simulink model "MappedCornerStiffness"  (R2021a)
settings: Solver=VariableStepAuto  StartTime=0.0  StopTime=15  RelTol=1e-3
values from neighbouring files (symbols this model uses):
  Ts = 0.05    [controller_setup.m]    (also in test.m = 0.1)
libraries: autolibshared x4
settings Model: Creator=chnwa  LastModifiedBy=chnwa

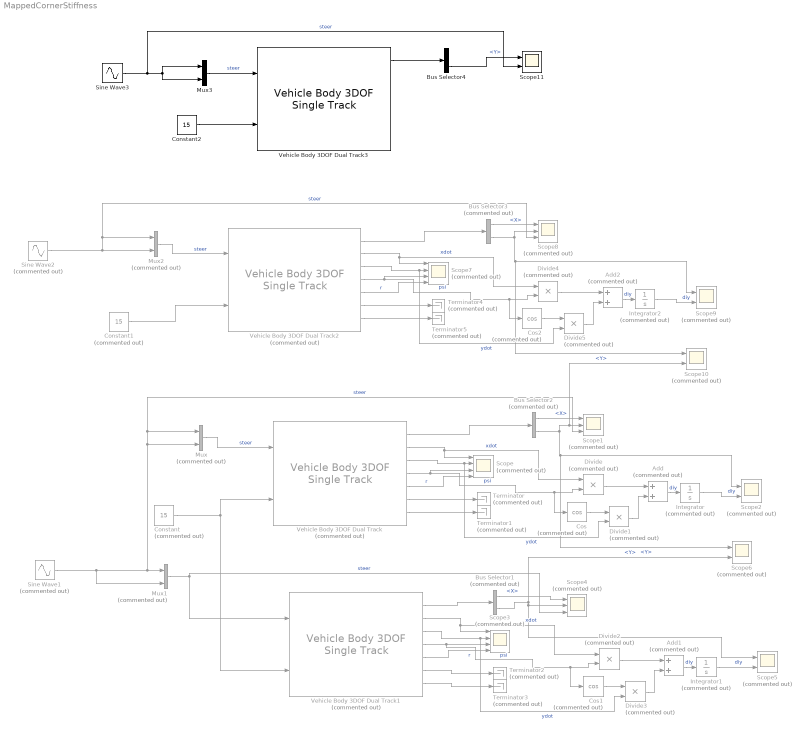
== system MappedCornerStiffness ==
  Add : Sum  Commented=on
  Add1 : Sum  Commented=on
  Add2 : Sum  Commented=on
  Bus Selector1 : BusSelector  Commented=on  OutputSignals=InertFrm.Cg.Disp.X,InertFrm.Cg.Disp.Y
  Bus Selector2 : BusSelector  Commented=on  OutputSignals=InertFrm.Cg.Disp.X,InertFrm.Cg.Disp.Y
  Bus Selector3 : BusSelector  Commented=on  OutputSignals=InertFrm.Cg.Disp.X,InertFrm.Cg.Disp.Y
  Bus Selector4 : BusSelector  OutputSignals=InertFrm.Cg.Disp.X,InertFrm.Cg.Disp.Y
  Constant : Constant  Commented=on  Value=15
  Constant1 : Constant  Commented=on  Value=15
  Constant2 : Constant  Value=15
  Cos : Trigonometry  Commented=on  Operator=cos
  Cos1 : Trigonometry  Commented=on  Operator=cos
  Cos2 : Trigonometry  Commented=on  Operator=cos
  Divide{,1..5} (6 alike) : Product  Commented=on  Inputs=**
  Integrator : Integrator  Commented=on
  Integrator1 : Integrator  Commented=on
  Integrator2 : Integrator  Commented=on
  Mux : Mux  Commented=on  Inputs=2
  Mux1 : Mux  Commented=on  Inputs=2
  Mux2 : Mux  Commented=on  Inputs=2
  Mux3 : Mux  Inputs=2
  Scope : Scope  Commented=on  NumInputPorts=4
  Scope1 : Scope  Commented=on  NumInputPorts=3
  Scope{2,5..6,9..10} (5 alike) : Scope  Commented=on  NumInputPorts=2
  Scope11 : Scope  NumInputPorts=2
  Scope3 : Scope  Commented=on  NumInputPorts=4
  Scope4 : Scope  Commented=on  NumInputPorts=3
  Scope7 : Scope  Commented=on  NumInputPorts=4
  Scope8 : Scope  Commented=on  NumInputPorts=3
  Sine Wave1 : Sin  Commented=on  Amplitude=0.01  Frequency=pi/5  SampleTime=Ts
  Sine Wave2 : Sin  Commented=on  Amplitude=-0.01  Frequency=pi/5  SampleTime=Ts
  Sine Wave3 : Sin  Amplitude=-0.01  Frequency=pi/15  SampleTime=Ts
  Terminator{,1..5} (6 alike) : Terminator  Commented=on
  Vehicle Body 3DOF Dual Track : autolibshared/Vehicle Body 3DOF Single Track  Commented=on  trackMode=Dual  inputMode=External longitudinal velocity  frontSteerMode=on  rearSteerMode=off  windMode=off  muMode=off  extFMode=off  extMMode=off  htchFMode=off  htchMMode=off  extXo=off  extpsio=off  extxdoto=off  extro=off  extYo=off  extTamb=off  extydoto=off  aMode=2  NF=2  NR=2  m=2272  a=1.11  b=1.67  h=0.35  dh=1  hh=0.2  X_o=0  xdot_o=15  CalphaMode=off  sigmaMode=on  d=0  hl=0  w=[1.4,1.4]  Cy_f=13e4  Cy_r=13e4  sigma_f=.1  sigma_r=.1  alpha_f_brk=[-.1 .1]  Cy_f_data=[-1.3e5 1.3e5]  alpha_r_brk=[-.1 .1]  Cy_r_data=[-1.3e5 1.3e5]  Y_o=0  ydot_o=0  Izz=4600  psi_o=0  r_o=0  Af=2  Cd=.3  Cl=.1  Cpm=.1  beta_w=[0:0.01:0.3]  Cs=[0:0.03:0.9]  Cym=[0:0.01:0.3]  Pabs=101325  Tair=273  g=9.81  mu=1  xdot_tol=.01  Fznom=5000  Fxtire_sat=7e4  Fytire_sat=7e4  longOff=0  latOff=0  vertOff=0  wrapAng=off
      settings: SourceProductBaseCode=PW,DR,MT,UV,VE
  Vehicle Body 3DOF Dual Track1 : autolibshared/Vehicle Body 3DOF Single Track  Commented=on  trackMode=Dual  inputMode=External longitudinal velocity  frontSteerMode=on  rearSteerMode=off  windMode=off  muMode=off  extFMode=off  extMMode=off  htchFMode=off  htchMMode=off  extXo=off  extpsio=off  extxdoto=off  extro=off  extYo=off  extTamb=off  extydoto=off  aMode=2  NF=2  NR=2  m=2272  a=1.11  b=1.67  h=0.35  dh=1  hh=0.2  X_o=0  xdot_o=15  CalphaMode=off  sigmaMode=on  d=0  hl=0  w=[1.4,1.4]  Cy_f=1.3e5  Cy_r=1.3e5  sigma_f=.1  sigma_r=.1  alpha_f_brk=[-.1 .1]  Cy_f_data=[1.3e5 -1.3e5]  alpha_r_brk=[-.1 .1]  Cy_r_data=[1.3e5 -1.3e5]  Y_o=0  ydot_o=0  Izz=4600  psi_o=0  r_o=0  Af=2  Cd=.3  Cl=.1  Cpm=.1  beta_w=[0:0.01:0.3]  Cs=[0:0.03:0.9]  Cym=[0:0.01:0.3]  Pabs=101325  Tair=273  g=9.81  mu=1  xdot_tol=.01  Fznom=5000  Fxtire_sat=7e4  Fytire_sat=7e4  longOff=0  latOff=0  vertOff=0  wrapAng=off
      settings: SourceProductBaseCode=PW,DR,MT,UV,VE
  Vehicle Body 3DOF Dual Track2 : autolibshared/Vehicle Body 3DOF Single Track  Commented=on  trackMode=Dual  inputMode=External longitudinal velocity  frontSteerMode=on  rearSteerMode=off  windMode=off  muMode=off  extFMode=off  extMMode=off  htchFMode=off  htchMMode=off  extXo=off  extpsio=off  extxdoto=off  extro=off  extYo=off  extTamb=off  extydoto=off  aMode=2  NF=2  NR=2  m=2272  a=1.11  b=1.67  h=0.35  dh=1  hh=0.2  X_o=0  xdot_o=15  CalphaMode=off  sigmaMode=on  d=0  hl=0  w=[1.4,1.4]  Cy_f=13e4  Cy_r=13e4  sigma_f=.1  sigma_r=.1  alpha_f_brk=[-.1 .1]  Cy_f_data=[-1.3e5 1.3e5]  alpha_r_brk=[-.1 .1]  Cy_r_data=[-1.3e5 1.3e5]  Y_o=0  ydot_o=0  Izz=4600  psi_o=0  r_o=0  Af=2  Cd=.3  Cl=.1  Cpm=.1  beta_w=[0:0.01:0.3]  Cs=[0:0.03:0.9]  Cym=[0:0.01:0.3]  Pabs=101325  Tair=273  g=9.81  mu=1  xdot_tol=.01  Fznom=5000  Fxtire_sat=7e4  Fytire_sat=7e4  longOff=0  latOff=0  vertOff=0  wrapAng=off
      settings: SourceProductBaseCode=PW,DR,MT,UV,VE
  Vehicle Body 3DOF Dual Track3 : autolibshared/Vehicle Body 3DOF Single Track  trackMode=Dual  inputMode=External longitudinal velocity  frontSteerMode=on  rearSteerMode=off  windMode=off  muMode=off  extFMode=off  extMMode=off  htchFMode=off  htchMMode=off  extXo=off  extpsio=off  extxdoto=off  extro=off  extYo=off  extTamb=off  extydoto=off  aMode=2  NF=2  NR=2  m=2000  a=1.4  b=1.6  h=0.35  dh=1  hh=0.2  X_o=0  xdot_o=0  CalphaMode=on  sigmaMode=on  d=0  hl=0  w=[1.4,1.4]  Cy_f=12e3  Cy_r=11e3  sigma_f=.1  sigma_r=.1  alpha_f_brk=[-.1 .1]  Cy_f_data=[-9e3 9e3]  alpha_r_brk=[-.1 .1]  Cy_r_data=[-9e3 9e3]  Y_o=0  ydot_o=0  Izz=4000  psi_o=0  r_o=0  Af=2  Cd=.3  Cl=.1  Cpm=.1  beta_w=[0:0.01:0.3]  Cs=[0:0.03:0.9]  Cym=[0:0.01:0.3]  Pabs=101325  Tair=273  g=9.81  mu=1  xdot_tol=.01  Fznom=5000  Fxtire_sat=7e4  Fytire_sat=7e4  longOff=0  latOff=0  vertOff=0  wrapAng=off
      settings: SourceProductBaseCode=PW,DR,MT,UV,VE
  wires:
  Vehicle Body 3DOF Dual Track/2 -> Divide/1, Scope/1  "xdot"
  Vehicle Body 3DOF Dual Track/3 -> Divide1/2, Scope/2  "ydot"
  Vehicle Body 3DOF Dual Track/4 -> Cos/1, Divide/2, Scope/3  "psi"
  Vehicle Body 3DOF Dual Track/5 -> Scope/4  "r"
  Vehicle Body 3DOF Dual Track/6 -> Terminator/1
  Vehicle Body 3DOF Dual Track/7 -> Terminator1/1
  Divide/1 -> Add/1
  Cos/1 -> Divide1/1
  Divide1/1 -> Add/2
  Add/1 -> Integrator/1  "diy"
  Integrator/1 -> Scope2/2  "diy"
  Divide2/1 -> Add1/1
  Divide3/1 -> Add1/2
  Add1/1 -> Integrator1/1  "diy"
  Vehicle Body 3DOF Dual Track1/5 -> Scope3/4  "r"
  Vehicle Body 3DOF Dual Track1/4 -> Cos1/1, Divide2/2, Scope3/3  "psi"
  Vehicle Body 3DOF Dual Track1/7 -> Terminator3/1
  Bus Selector1/1 -> Scope4/1  "<X>"
  Integrator1/1 -> Scope5/2  "diy"
  Vehicle Body 3DOF Dual Track1/6 -> Terminator2/1
  Vehicle Body 3DOF Dual Track1/3 -> Divide3/2, Scope3/2  "ydot"
  Bus Selector1/2 -> Scope5/1, Scope4/2, Scope6/2  "<Y>"
  Mux/1 -> Vehicle Body 3DOF Dual Track/1  "steer"
  Vehicle Body 3DOF Dual Track1/1 -> Bus Selector1/1
  Vehicle Body 3DOF Dual Track1/2 -> Divide2/1, Scope3/1  "xdot"
  Cos1/1 -> Divide3/1
  Constant/1 -> Vehicle Body 3DOF Dual Track1/2, Vehicle Body 3DOF Dual Track/2
  Mux1/1 -> Scope4/3, Vehicle Body 3DOF Dual Track1/1  "steer"
  Sine Wave1/1 -> Mux/2, Scope1/3, Mux/1, Mux1/1, Mux1/2  "steer"
  Vehicle Body 3DOF Dual Track/1 -> Bus Selector2/1
  Bus Selector2/1 -> Scope1/1  "<X>"
  Bus Selector3/1 -> Scope8/1  "<X>"
  Integrator2/1 -> Scope9/2  "diy"
  Bus Selector3/2 -> Scope10/1, Scope9/1, Scope8/2  "<Y>"
  Vehicle Body 3DOF Dual Track2/1 -> Bus Selector3/1
  Constant1/1 -> Vehicle Body 3DOF Dual Track2/2
  Vehicle Body 3DOF Dual Track2/3 -> Divide5/2, Scope7/2  "ydot"
  Bus Selector2/2 -> Scope10/2, Scope1/2, Scope6/1, Scope2/1  "<Y>"
  Vehicle Body 3DOF Dual Track2/2 -> Divide4/1, Scope7/1  "xdot"
  Vehicle Body 3DOF Dual Track2/7 -> Terminator5/1
  Mux2/1 -> Vehicle Body 3DOF Dual Track2/1  "steer"
  Vehicle Body 3DOF Dual Track2/6 -> Terminator4/1
  Cos2/1 -> Divide5/1
  Divide5/1 -> Add2/2
  Vehicle Body 3DOF Dual Track2/4 -> Cos2/1, Divide4/2, Scope7/3  "psi"
  Divide4/1 -> Add2/1
  Vehicle Body 3DOF Dual Track2/5 -> Scope7/4  "r"
  Add2/1 -> Integrator2/1  "diy"
  Sine Wave2/1 -> Mux2/2, Scope8/3, Mux2/1  "steer"
  Constant2/1 -> Vehicle Body 3DOF Dual Track3/2
  Sine Wave3/1 -> Scope11/2, Mux3/1, Mux3/2  "steer"
  Vehicle Body 3DOF Dual Track3/1 -> Bus Selector4/1
  Bus Selector4/2 -> Scope11/1  "<Y>"
  Mux3/1 -> Vehicle Body 3DOF Dual Track3/1  "steer"
